simulink subsystem "s0330_switching_policy2"  (R2019b)
settings: Solver=VariableStepAuto  StartTime=0.0  StopTime=10.0  RelTol=1e-3
undefined symbols (not defined in the file): __PRM__SERIALIZED__DATA__, SubsystemReferenceBlock
settings Model: Creator=paolo  LastModifiedBy=alessandro

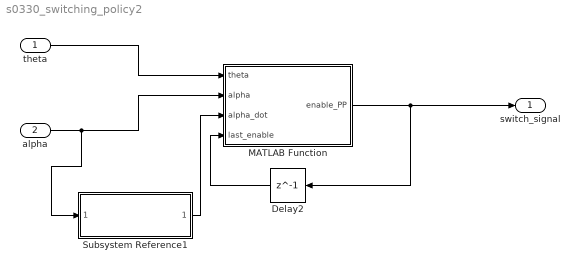
== system s0330_switching_policy2 ==
  theta : Inport
  alpha : Inport  Port=2
  Delay2 : Delay  DelayLength=1  InitialCondition=false
  MATLAB Function : MATLAB Function  TreatAsAtomicUnit=on
  Subsystem Reference1 : Subsystem  BlockKeywords=__PRM__SERIALIZED__DATA__:SubsystemReferenceBlock  ReferencedSubsystem=Filtered_Derivative  num=num_der_filter  den=den_der_filter
  switch_signal : Outport
  wires:
  theta/1 -> MATLAB Function/1(theta)
  alpha/1 -> MATLAB Function/2(alpha), Subsystem Reference1/1
  MATLAB Function/1(enable_PP) -> Delay2/1, switch_signal/1
  Delay2/1 -> MATLAB Function/4(last_enable)
  Subsystem Reference1/1 -> MATLAB Function/3(alpha_dot)

== matlab function s0330_switching_policy2/MATLAB Function ==
  data: theta input; enable_PP output; alpha input; alpha_dot input; last_enable input boolean
function enable_PP = PP_enabler(theta, alpha, alpha_dot, last_enable)

alpha_diff = alpha*180/pi - 180;
theta = theta*180/pi;

stop_condition = false;
while ~stop_condition
    if alpha_diff > 180
        alpha_diff = alpha_diff - 360;
    elseif alpha_diff < -180
        alpha_diff = alpha_diff + 360;
    else
        stop_condition = true;
    end
end

if (abs(alpha_diff) < 15 && abs(alpha_dot) < 1 && abs(theta) < 90) || last_enable
    enable_PP = true;
else
    enable_PP = false;
end

end
